simulink model "IEEE30_case"  (R2024b)
settings: Solver=FixedStepAuto  StartTime=0  StopTime=5  FixedStep=1e-7  RelTol=1e-3
values from neighbouring files (symbols this model uses):
  GFL_DFIG_7_C_bus = 0.08    [IEEE30_case_parameters.m]
  GFL_DFIG_7_D_mutual = 2.500000e+3    (= 2500)    [IEEE30_case_parameters.m]
  GFL_DFIG_7_f0 = 60    [IEEE30_case_parameters.m]
  GFL_DFIG_7_gPLLi = 3200    [IEEE30_case_parameters.m]
  GFL_DFIG_7_gPLLp = 650    [IEEE30_case_parameters.m]
  GFL_DFIG_7_H_WT = 0.4    [IEEE30_case_parameters.m]
  GFL_DFIG_7_Hg = 0.8    [IEEE30_case_parameters.m]
  GFL_DFIG_7_Igq_ref = 0    [IEEE30_case_parameters.m]
  GFL_DFIG_7_Ird_ref = 704.45696    [IEEE30_case_parameters.m]
  GFL_DFIG_7_KI_V = -300000    [IEEE30_case_parameters.m]
  GFL_DFIG_7_KP_V = -1000    [IEEE30_case_parameters.m]
  GFL_DFIG_7_Ksh = 1.254300e+4    (= 12543)    [IEEE30_case_parameters.m]
  GFL_DFIG_7_Lg = 0.000483    [IEEE30_case_parameters.m]
  GFL_DFIG_7_Lm_pu = 4    [IEEE30_case_parameters.m]
  GFL_DFIG_7_N = 100    [IEEE30_case_parameters.m]
  GFL_DFIG_7_p = 2    [IEEE30_case_parameters.m]
  GFL_DFIG_7_Pitch = 0    [IEEE30_case_parameters.m]
  GFL_DFIG_7_R = 44    [IEEE30_case_parameters.m]
  GFL_DFIG_7_Rg = 2.000000e-5    (= 2e-05)    [IEEE30_case_parameters.m]
  GFL_DFIG_7_rho = 1.225    [IEEE30_case_parameters.m]
  GFL_DFIG_7_rPLLi = 4500    [IEEE30_case_parameters.m]
  GFL_DFIG_7_rPLLp = 620    [IEEE30_case_parameters.m]
  GFL_DFIG_7_Rs_pu = 0.011    [IEEE30_case_parameters.m]
  GFL_DFIG_7_Sbase = 2.000000e+6    (= 2000000)    [IEEE30_case_parameters.m]
  GFL_DFIG_7_ugq_ref = 0    [IEEE30_case_parameters.m]
  GFL_DFIG_7_usd_ref = 0    [IEEE30_case_parameters.m]
  GFL_DFIG_7_Vbase = 690    [IEEE30_case_parameters.m]
  GFL_DFIG_7_Vdc_ref = 1200    [IEEE30_case_parameters.m]
  GFL_DFIG_7_wind = 12    [IEEE30_case_parameters.m]
  GFL_DFIG_7_wm_ref = 518.184209    [IEEE30_case_parameters.m]
  SG_D_13_D = 0.01056    [IEEE30_case_parameters.m]
  SG_D_13_EnableSaturation = 0    [IEEE30_case_parameters.m]
  SG_D_13_f0 = 60    [IEEE30_case_parameters.m]
  SG_D_13_H = 7.5    [IEEE30_case_parameters.m]
  SG_D_13_K_A = 20    [IEEE30_case_parameters.m]
  SG_D_13_K_E = 1.000000e+1    (= 10)    [IEEE30_case_parameters.m]
  SG_D_13_K_F = 2.363    [IEEE30_case_parameters.m]
  SG_D_13_K_s = 0.5    [IEEE30_case_parameters.m]
  SG_D_13_R_a = 0.001088    [IEEE30_case_parameters.m]
  SG_D_13_S_A = 1    [IEEE30_case_parameters.m]
  SG_D_13_S_B = 0.103    [IEEE30_case_parameters.m]
  SG_D_13_S_N = 10.659857    [IEEE30_case_parameters.m]
  SG_D_13_SpeedPara = 200    [IEEE30_case_parameters.m]
  SG_D_13_T_0 = 0.370163    [IEEE30_case_parameters.m]
  SG_D_13_T_1 = 0.3    [IEEE30_case_parameters.m]
  SG_D_13_T_2 = 0.05    [IEEE30_case_parameters.m]
  SG_D_13_T_3 = 0.02    [IEEE30_case_parameters.m]
  SG_D_13_T_4 = 0.005    [IEEE30_case_parameters.m]
  SG_D_13_T_A = 0.02    [IEEE30_case_parameters.m]
  SG_D_13_T_dd = 8.000000e+0    (= 8)    [IEEE30_case_parameters.m]
  SG_D_13_T_ddd = 0.04    [IEEE30_case_parameters.m]
  SG_D_13_T_E = 0.314    [IEEE30_case_parameters.m]
  SG_D_13_T_F = 0.35    [IEEE30_case_parameters.m]
  SG_D_13_T_qd = 0.8    [IEEE30_case_parameters.m]
  SG_D_13_T_qdd = 0.02    [IEEE30_case_parameters.m]
  SG_D_13_T_speed = 0.1    [IEEE30_case_parameters.m]
  SG_D_13_T_w = 0.5    [IEEE30_case_parameters.m]
  SG_D_13_V_ref = 1.696619    [IEEE30_case_parameters.m]
  SG_D_13_w_ref = 376.991118    [IEEE30_case_parameters.m]
  SG_D_13_x_d = 1.9    [IEEE30_case_parameters.m]
  SG_D_13_x_dd = 0.302    [IEEE30_case_parameters.m]
  SG_D_13_x_ddd = 0.204    [IEEE30_case_parameters.m]
  SG_D_13_x_l = 0.05    [IEEE30_case_parameters.m]
  SG_D_13_x_q = 1.3    [IEEE30_case_parameters.m]
  SG_D_13_x_qd = 0.5    [IEEE30_case_parameters.m]
  SG_D_13_x_qdd = 0.3    [IEEE30_case_parameters.m]
  SG_D_1_D = 0.01056    [IEEE30_case_parameters.m]
  SG_D_1_EnableSaturation = 0    [IEEE30_case_parameters.m]
  SG_D_1_f0 = 60    [IEEE30_case_parameters.m]
  SG_D_1_H = 7.5    [IEEE30_case_parameters.m]
  SG_D_1_K_A = 20    [IEEE30_case_parameters.m]
  SG_D_1_K_E = 1.000000e+1    (= 10)    [IEEE30_case_parameters.m]
  SG_D_1_K_F = 2.363    [IEEE30_case_parameters.m]
  SG_D_1_K_s = 0.5    [IEEE30_case_parameters.m]
  SG_D_1_R_a = 0.001088    [IEEE30_case_parameters.m]
  SG_D_1_S_A = 1    [IEEE30_case_parameters.m]
  SG_D_1_S_B = 0.103    [IEEE30_case_parameters.m]
  SG_D_1_S_N = 10.659857    [IEEE30_case_parameters.m]
  SG_D_1_SpeedPara = 200    [IEEE30_case_parameters.m]
  SG_D_1_T_0 = 0.259812    [IEEE30_case_parameters.m]
  SG_D_1_T_1 = 0.3    [IEEE30_case_parameters.m]
  SG_D_1_T_2 = 0.05    [IEEE30_case_parameters.m]
  SG_D_1_T_3 = 0.02    [IEEE30_case_parameters.m]
  SG_D_1_T_4 = 0.005    [IEEE30_case_parameters.m]
  SG_D_1_T_A = 0.02    [IEEE30_case_parameters.m]
  SG_D_1_T_dd = 8.000000e+0    (= 8)    [IEEE30_case_parameters.m]
  SG_D_1_T_ddd = 0.04    [IEEE30_case_parameters.m]
  SG_D_1_T_E = 0.314    [IEEE30_case_parameters.m]
  SG_D_1_T_F = 0.35    [IEEE30_case_parameters.m]
  SG_D_1_T_qd = 0.8    [IEEE30_case_parameters.m]
  SG_D_1_T_qdd = 0.02    [IEEE30_case_parameters.m]
  SG_D_1_T_speed = 0.1    [IEEE30_case_parameters.m]
  SG_D_1_T_w = 0.5    [IEEE30_case_parameters.m]
  SG_D_1_V_ref = 1.544107    [IEEE30_case_parameters.m]
  SG_D_1_w_ref = 376.991118    [IEEE30_case_parameters.m]
  SG_D_1_x_d = 1.9    [IEEE30_case_parameters.m]
  SG_D_1_x_dd = 0.302    [IEEE30_case_parameters.m]
  SG_D_1_x_ddd = 0.204    [IEEE30_case_parameters.m]
  SG_D_1_x_l = 0.05    [IEEE30_case_parameters.m]
  SG_D_1_x_q = 1.3    [IEEE30_case_parameters.m]
  SG_D_1_x_qd = 0.5    [IEEE30_case_parameters.m]
  SG_D_1_x_qdd = 0.3    [IEEE30_case_parameters.m]
  SG_D_22_D = 0.01056    [IEEE30_case_parameters.m]
  SG_D_22_EnableSaturation = 0    [IEEE30_case_parameters.m]
  SG_D_22_f0 = 60    [IEEE30_case_parameters.m]
  SG_D_22_H = 7.5    [IEEE30_case_parameters.m]
  SG_D_22_K_A = 20    [IEEE30_case_parameters.m]
  SG_D_22_K_E = 1.000000e+1    (= 10)    [IEEE30_case_parameters.m]
  SG_D_22_K_F = 2.363    [IEEE30_case_parameters.m]
  SG_D_22_K_s = 0.5    [IEEE30_case_parameters.m]
  SG_D_22_R_a = 0.001088    [IEEE30_case_parameters.m]
  SG_D_22_S_A = 1    [IEEE30_case_parameters.m]
  SG_D_22_S_B = 0.103    [IEEE30_case_parameters.m]
  SG_D_22_S_N = 10.659857    [IEEE30_case_parameters.m]
  SG_D_22_SpeedPara = 200    [IEEE30_case_parameters.m]
  SG_D_22_T_0 = 0.216121    [IEEE30_case_parameters.m]
  SG_D_22_T_1 = 0.3    [IEEE30_case_parameters.m]
  SG_D_22_T_2 = 0.05    [IEEE30_case_parameters.m]
  SG_D_22_T_3 = 0.02    [IEEE30_case_parameters.m]
  SG_D_22_T_4 = 0.005    [IEEE30_case_parameters.m]
  ... (+126 more)
(part 5 of 27)

== system IEEE30_case/AC_1/d_id_line_12_15_block ==
  note: d_id_line_12_15 in IEEE30_case
      | $376.991118430775\,\mathrm{iq}_{\mathrm{line},12,15}-202.995217616571\,\mathrm{id}_{\mathrm{line},12,15}+2899.93168023673\,\mathrm{vd}_{\mathrm{bus},12}-2899.93168023673\,\mathrm{vd}_{\mathrm{bus},15}$
      | Automatically generated on 2025-11-01 18:41:36 .
  State_id_line_12_15_19cb2 : Inport
  State_iq_line_12_15_08071 : Inport  Port=2
  State_vd_bus_12_a4ba8 : Inport  Port=3
  State_vd_bus_15_2851a : Inport  Port=4
  Add_1c604 : Sum
  Add_88b54 : Sum
  Constant_-202.995217616571_6ff68 : Constant  Value=-202.995217616571
  Constant_2899.93168023673_4202a : Constant  Value=2899.93168023673
  Constant_2899.93168023673_fe615 : Constant  Value=2899.93168023673
  Constant_376.991118430775_4d075 : Constant  Value=376.991118430775
  Product_04dd2 : Product
  Product_066f0 : Product
  Product_6a2b6 : Product
  Product_79b71 : Product
  Subtract_280ce : Sum  Inputs=+-
  Blockout_d_id_line_12_15_9a1c2 : Outport
  wires:
  State_id_line_12_15_19cb2/1 -> Product_04dd2/2
  Constant_-202.995217616571_6ff68/1 -> Product_04dd2/1
  Constant_376.991118430775_4d075/1 -> Product_79b71/1
  Product_6a2b6/1 -> Add_1c604/2
  Constant_2899.93168023673_fe615/1 -> Product_6a2b6/1
  State_iq_line_12_15_08071/1 -> Product_79b71/2
  Product_79b71/1 -> Add_88b54/2
  Product_04dd2/1 -> Add_88b54/1
  State_vd_bus_12_a4ba8/1 -> Product_6a2b6/2
  Add_88b54/1 -> Add_1c604/1
  Product_066f0/1 -> Subtract_280ce/2
  Constant_2899.93168023673_4202a/1 -> Product_066f0/1
  State_vd_bus_15_2851a/1 -> Product_066f0/2
  Add_1c604/1 -> Subtract_280ce/1
  Subtract_280ce/1 -> Blockout_d_id_line_12_15_9a1c2/1

== system IEEE30_case/AC_1/d_id_line_12_16_block ==
  note: d_id_line_12_16 in IEEE30_case
      | $376.991118430775\,\mathrm{iq}_{\mathrm{line},12,16}-169.646003293849\,\mathrm{id}_{\mathrm{line},12,16}+1884.95559215388\,\mathrm{vd}_{\mathrm{bus},12}-1884.95559215388\,\mathrm{vd}_{\mathrm{bus},16}$
      | Automatically generated on 2025-11-01 18:41:38 .
  State_id_line_12_16_8024a : Inport
  State_iq_line_12_16_288fb : Inport  Port=2
  State_vd_bus_12_31adb : Inport  Port=3
  State_vd_bus_16_dfe3f : Inport  Port=4
  Add_7fa9a : Sum
  Add_82f4b : Sum
  Constant_-169.646003293849_e986b : Constant  Value=-169.646003293849
  Constant_1884.95559215388_c1875 : Constant  Value=1884.95559215388
  Constant_1884.95559215388_da5ce : Constant  Value=1884.95559215388
  Constant_376.991118430775_e57b6 : Constant  Value=376.991118430775
  Product_08c30 : Product
  Product_0c215 : Product
  Product_538c2 : Product
  Product_ba034 : Product
  Subtract_28196 : Sum  Inputs=+-
  Blockout_d_id_line_12_16_004d6 : Outport
  wires:
  Constant_-169.646003293849_e986b/1 -> Product_08c30/1
  Constant_376.991118430775_e57b6/1 -> Product_538c2/1
  Product_538c2/1 -> Add_82f4b/2
  State_id_line_12_16_8024a/1 -> Product_08c30/2
  State_iq_line_12_16_288fb/1 -> Product_538c2/2
  Product_08c30/1 -> Add_82f4b/1
  Constant_1884.95559215388_c1875/1 -> Product_ba034/1
  State_vd_bus_12_31adb/1 -> Product_ba034/2
  Add_82f4b/1 -> Add_7fa9a/1
  Product_ba034/1 -> Add_7fa9a/2
  Product_0c215/1 -> Subtract_28196/2
  Constant_1884.95559215388_da5ce/1 -> Product_0c215/1
  State_vd_bus_16_dfe3f/1 -> Product_0c215/2
  Add_7fa9a/1 -> Subtract_28196/1
  Subtract_28196/1 -> Blockout_d_id_line_12_16_004d6/1

== system IEEE30_case/AC_1/d_id_line_14_15_block ==
  note: d_id_line_14_15 in IEEE30_case
      | $376.991118430775\,\mathrm{iq}_{\mathrm{line},14,15}-414.690230273853\,\mathrm{id}_{\mathrm{line},14,15}+1884.95559215388\,\mathrm{vd}_{\mathrm{bus},14}-1884.95559215388\,\mathrm{vd}_{\mathrm{bus},15}$
      | Automatically generated on 2025-11-01 18:41:40 .
  State_id_line_14_15_28cb1 : Inport
  State_iq_line_14_15_9579a : Inport  Port=2
  State_vd_bus_14_5ffe4 : Inport  Port=3
  State_vd_bus_15_c6d58 : Inport  Port=4
  Add_03647 : Sum
  Add_442a9 : Sum
  Constant_-414.690230273853_aa946 : Constant  Value=-414.690230273853
  Constant_1884.95559215388_3e1ac : Constant  Value=1884.95559215388
  Constant_1884.95559215388_7cbb8 : Constant  Value=1884.95559215388
  Constant_376.991118430775_5b540 : Constant  Value=376.991118430775
  Product_16522 : Product
  Product_81fd4 : Product
  Product_9c15a : Product
  Product_c85a0 : Product
  Subtract_fac3d : Sum  Inputs=+-
  Blockout_d_id_line_14_15_f4e19 : Outport
  wires:
  Product_c85a0/1 -> Add_03647/1
  Constant_-414.690230273853_aa946/1 -> Product_c85a0/1
  State_id_line_14_15_28cb1/1 -> Product_c85a0/2
  Constant_376.991118430775_5b540/1 -> Product_16522/1
  Product_16522/1 -> Add_03647/2
  State_iq_line_14_15_9579a/1 -> Product_16522/2
  Product_9c15a/1 -> Add_442a9/2
  Constant_1884.95559215388_3e1ac/1 -> Product_9c15a/1
  State_vd_bus_14_5ffe4/1 -> Product_9c15a/2
  Add_03647/1 -> Add_442a9/1
  Product_81fd4/1 -> Subtract_fac3d/2
  Constant_1884.95559215388_7cbb8/1 -> Product_81fd4/1
  State_vd_bus_15_c6d58/1 -> Product_81fd4/2
  Add_442a9/1 -> Subtract_fac3d/1
  Subtract_fac3d/1 -> Blockout_d_id_line_14_15_f4e19/1

== system IEEE30_case/AC_1/d_id_line_15_18_block ==
  note: d_id_line_15_18 in IEEE30_case
      | $376.991118430775\,\mathrm{iq}_{\mathrm{line},15,18}-188.495559215388\,\mathrm{id}_{\mathrm{line},15,18}+1713.59599286716\,\mathrm{vd}_{\mathrm{bus},15}-1713.59599286716\,\mathrm{vd}_{\mathrm{bus},18}$
      | Automatically generated on 2025-11-01 18:41:45 .
  State_id_line_15_18_9ff35 : Inport
  State_iq_line_15_18_872e9 : Inport  Port=2
  State_vd_bus_15_67b4c : Inport  Port=3
  State_vd_bus_18_e7afb : Inport  Port=4
  Add_4abb7 : Sum
  Add_ea80a : Sum
  Constant_-188.495559215388_eae43 : Constant  Value=-188.495559215388
  Constant_1713.59599286716_37fdf : Constant  Value=1713.59599286716
  Constant_1713.59599286716_e4c6f : Constant  Value=1713.59599286716
  Constant_376.991118430775_f78d8 : Constant  Value=376.991118430775
  Product_a3e74 : Product
  Product_c991e : Product
  Product_e914a : Product
  Product_ea7c3 : Product
  Subtract_e5fa3 : Sum  Inputs=+-
  Blockout_d_id_line_15_18_32fdd : Outport
  wires:
  Constant_-188.495559215388_eae43/1 -> Product_ea7c3/1
  Constant_376.991118430775_f78d8/1 -> Product_a3e74/1
  State_id_line_15_18_9ff35/1 -> Product_ea7c3/2
  Product_a3e74/1 -> Add_ea80a/2
  State_iq_line_15_18_872e9/1 -> Product_a3e74/2
  Product_ea7c3/1 -> Add_ea80a/1
  State_vd_bus_15_67b4c/1 -> Product_c991e/2
  Product_c991e/1 -> Add_4abb7/2
  Constant_1713.59599286716_e4c6f/1 -> Product_c991e/1
  Add_ea80a/1 -> Add_4abb7/1
  Product_e914a/1 -> Subtract_e5fa3/2
  Constant_1713.59599286716_37fdf/1 -> Product_e914a/1
  State_vd_bus_18_e7afb/1 -> Product_e914a/2
  Add_4abb7/1 -> Subtract_e5fa3/1
  Subtract_e5fa3/1 -> Blockout_d_id_line_15_18_32fdd/1

== system IEEE30_case/AC_1/d_id_line_15_23_block ==
  note: d_id_line_15_23 in IEEE30_case
      | $376.991118430775\,\mathrm{iq}_{\mathrm{line},15,23}-188.495559215388\,\mathrm{id}_{\mathrm{line},15,23}+1884.95559215388\,\mathrm{vd}_{\mathrm{bus},15}-1884.95559215388\,\mathrm{vd}_{\mathrm{bus},23}$
      | Automatically generated on 2025-11-01 18:42:03 .
  State_id_line_15_23_5b9f7 : Inport
  State_iq_line_15_23_b33ff : Inport  Port=2
  State_vd_bus_15_742a0 : Inport  Port=3
  State_vd_bus_23_ce9b8 : Inport  Port=4
  Add_304c8 : Sum
  Add_d6195 : Sum
  Constant_-188.495559215388_5b43b : Constant  Value=-188.495559215388
  Constant_1884.95559215388_346b1 : Constant  Value=1884.95559215388
  Constant_1884.95559215388_64cf3 : Constant  Value=1884.95559215388
  Constant_376.991118430775_82cf8 : Constant  Value=376.991118430775
  Product_18461 : Product
  Product_35b29 : Product
  Product_4bfc7 : Product
  Product_954db : Product
  Subtract_3f90f : Sum  Inputs=+-
  Blockout_d_id_line_15_23_c2a70 : Outport
  wires:
  Constant_-188.495559215388_5b43b/1 -> Product_35b29/1
  State_id_line_15_23_5b9f7/1 -> Product_35b29/2
  Constant_376.991118430775_82cf8/1 -> Product_4bfc7/1
  State_iq_line_15_23_b33ff/1 -> Product_4bfc7/2
  Product_4bfc7/1 -> Add_304c8/2
  Product_35b29/1 -> Add_304c8/1
  Product_18461/1 -> Add_d6195/2
  Constant_1884.95559215388_64cf3/1 -> Product_18461/1
  State_vd_bus_15_742a0/1 -> Product_18461/2
  Add_304c8/1 -> Add_d6195/1
  Product_954db/1 -> Subtract_3f90f/2
  Constant_1884.95559215388_346b1/1 -> Product_954db/1
  State_vd_bus_23_ce9b8/1 -> Product_954db/2
  Add_d6195/1 -> Subtract_3f90f/1
  Subtract_3f90f/1 -> Blockout_d_id_line_15_23_c2a70/1

== system IEEE30_case/AC_1/d_id_line_16_17_block ==
  note: d_id_line_16_17 in IEEE30_case
      | $376.991118430775\,\mathrm{iq}_{\mathrm{line},16,17}-158.733102497168\,\mathrm{id}_{\mathrm{line},16,17}+1984.16378121461\,\mathrm{vd}_{\mathrm{bus},16}-1984.16378121461\,\mathrm{vd}_{\mathrm{bus},17}$
      | Automatically generated on 2025-11-01 18:41:43 .
  State_id_line_16_17_5c8bf : Inport
  State_iq_line_16_17_49d5c : Inport  Port=2
  State_vd_bus_16_c102f : Inport  Port=3
  State_vd_bus_17_81d16 : Inport  Port=4
  Add_48fb3 : Sum
  Add_527f8 : Sum
  Constant_-158.733102497168_b2c29 : Constant  Value=-158.733102497168
  Constant_1984.16378121461_03e4f : Constant  Value=1984.16378121461
  Constant_1984.16378121461_7c6ef : Constant  Value=1984.16378121461
  Constant_376.991118430775_1e0c9 : Constant  Value=376.991118430775
  Product_01cb9 : Product
  Product_0d51e : Product
  Product_5ed86 : Product
  Product_f72dc : Product
  Subtract_cb5b6 : Sum  Inputs=+-
  Blockout_d_id_line_16_17_1cf66 : Outport
  wires:
  Constant_-158.733102497168_b2c29/1 -> Product_f72dc/1
  Constant_376.991118430775_1e0c9/1 -> Product_01cb9/1
  Product_01cb9/1 -> Add_48fb3/2
  Product_f72dc/1 -> Add_48fb3/1
  State_id_line_16_17_5c8bf/1 -> Product_f72dc/2
  Product_0d51e/1 -> Add_527f8/2
  Constant_1984.16378121461_03e4f/1 -> Product_0d51e/1
  State_iq_line_16_17_49d5c/1 -> Product_01cb9/2
  State_vd_bus_16_c102f/1 -> Product_0d51e/2
  Add_48fb3/1 -> Add_527f8/1
  Constant_1984.16378121461_7c6ef/1 -> Product_5ed86/1
  Add_527f8/1 -> Subtract_cb5b6/1
  State_vd_bus_17_81d16/1 -> Product_5ed86/2
  Product_5ed86/1 -> Subtract_cb5b6/2
  Subtract_cb5b6/1 -> Blockout_d_id_line_16_17_1cf66/1

== system IEEE30_case/AC_1/d_id_line_18_19_block ==
  note: d_id_line_18_19 in IEEE30_case
      | $376.991118430775\,\mathrm{iq}_{\mathrm{line},18,19}-173.995900814204\,\mathrm{id}_{\mathrm{line},18,19}+2899.93168023673\,\mathrm{vd}_{\mathrm{bus},18}-2899.93168023673\,\mathrm{vd}_{\mathrm{bus},19}$
      | Automatically generated on 2025-11-01 18:41:47 .
  State_id_line_18_19_ee31e : Inport
  State_iq_line_18_19_bad0a : Inport  Port=2
  State_vd_bus_18_26e57 : Inport  Port=3
  State_vd_bus_19_37873 : Inport  Port=4
  Add_0bb69 : Sum
  Add_79b81 : Sum
  Constant_-173.995900814204_e40f3 : Constant  Value=-173.995900814204
  Constant_2899.93168023673_2d509 : Constant  Value=2899.93168023673
  Constant_2899.93168023673_80d84 : Constant  Value=2899.93168023673
  Constant_376.991118430775_81f31 : Constant  Value=376.991118430775
  Product_a93df : Product
  Product_b05af : Product
  Product_ca76e : Product
  Product_e4da4 : Product
  Subtract_630ad : Sum  Inputs=+-
  Blockout_d_id_line_18_19_39807 : Outport
  wires:
  State_id_line_18_19_ee31e/1 -> Product_a93df/2
  Constant_-173.995900814204_e40f3/1 -> Product_a93df/1
  Constant_376.991118430775_81f31/1 -> Product_ca76e/1
  Product_ca76e/1 -> Add_0bb69/2
  State_iq_line_18_19_bad0a/1 -> Product_ca76e/2
  Product_a93df/1 -> Add_0bb69/1
  Add_0bb69/1 -> Add_79b81/1
  Constant_2899.93168023673_80d84/1 -> Product_b05af/1
  State_vd_bus_18_26e57/1 -> Product_b05af/2
  Product_b05af/1 -> Add_79b81/2
  Product_e4da4/1 -> Subtract_630ad/2
  Constant_2899.93168023673_2d509/1 -> Product_e4da4/1
  State_vd_bus_19_37873/1 -> Product_e4da4/2
  Add_79b81/1 -> Subtract_630ad/1
  Subtract_630ad/1 -> Blockout_d_id_line_18_19_39807/1

== system IEEE30_case/AC_1/d_id_line_19_20_block ==
  note: d_id_line_19_20 in IEEE30_case
      | $376.991118430775\,\mathrm{iq}_{\mathrm{line},19,20}-161.567622184618\,\mathrm{id}_{\mathrm{line},19,20}+5385.58740615393\,\mathrm{vd}_{\mathrm{bus},19}-5385.58740615393\,\mathrm{vd}_{\mathrm{bus},20}$
      | Automatically generated on 2025-11-01 18:41:49 .
  State_id_line_19_20_52ad5 : Inport
  State_iq_line_19_20_aecba : Inport  Port=2
  State_vd_bus_19_720ac : Inport  Port=3
  State_vd_bus_20_fc360 : Inport  Port=4
  Add_85617 : Sum
  Add_b55b6 : Sum
  Constant_-161.567622184618_669a2 : Constant  Value=-161.567622184618
  Constant_376.991118430775_79d8f : Constant  Value=376.991118430775
  Constant_5385.58740615393_4a1b5 : Constant  Value=5385.58740615393
  Constant_5385.58740615393_9f343 : Constant  Value=5385.58740615393
  Product_21136 : Product
  Product_39dca : Product
  Product_62d92 : Product
  Product_79959 : Product
  Subtract_e7c18 : Sum  Inputs=+-
  Blockout_d_id_line_19_20_50907 : Outport
  wires:
  State_vd_bus_19_720ac/1 -> Product_79959/2
  Constant_-161.567622184618_669a2/1 -> Product_21136/1
  Product_79959/1 -> Add_85617/2
  Constant_5385.58740615393_9f343/1 -> Product_79959/1
  Subtract_e7c18/1 -> Blockout_d_id_line_19_20_50907/1
  State_id_line_19_20_52ad5/1 -> Product_21136/2
  Constant_376.991118430775_79d8f/1 -> Product_39dca/1
  Product_39dca/1 -> Add_b55b6/2
  State_iq_line_19_20_aecba/1 -> Product_39dca/2
  Product_21136/1 -> Add_b55b6/1
  Add_b55b6/1 -> Add_85617/1
  Product_62d92/1 -> Subtract_e7c18/2
  Constant_5385.58740615393_4a1b5/1 -> Product_62d92/1
  State_vd_bus_20_fc360/1 -> Product_62d92/2
  Add_85617/1 -> Subtract_e7c18/1

== system IEEE30_case/AC_1/d_id_line_1_2_block ==
  note: d_id_line_1_2 in IEEE30_case
      | $376.991118430775\,\mathrm{iq}_{\mathrm{line},1,2}-125.663706143592\,\mathrm{id}_{\mathrm{line},1,2}+6283.18530717959\,\mathrm{vd}_{\mathrm{bus},1}-6283.18530717959\,\mathrm{vd}_{\mathrm{bus},2}$
      | Automatically generated on 2025-11-01 18:40:56 .
  State_id_line_1_2_ffdd4 : Inport
  State_iq_line_1_2_034b5 : Inport  Port=2
  State_vd_bus_1_c4c37 : Inport  Port=3
  State_vd_bus_2_3fb4b : Inport  Port=4
  Add_2f17b : Sum
  Add_58b2b : Sum
  Constant_-125.663706143592_1505d : Constant  Value=-125.663706143592
  Constant_376.991118430775_520bb : Constant  Value=376.991118430775
  Constant_6283.18530717959_4c671 : Constant  Value=6283.18530717959
  Constant_6283.18530717959_8a0e7 : Constant  Value=6283.18530717959
  Product_36a67 : Product
  Product_59a0b : Product
  Product_b8331 : Product
  Product_bf9d6 : Product
  Subtract_e7e69 : Sum  Inputs=+-
  Blockout_d_id_line_1_2_c33ff : Outport
  wires:
  Constant_-125.663706143592_1505d/1 -> Product_59a0b/1
  Product_59a0b/1 -> Add_58b2b/1
  State_id_line_1_2_ffdd4/1 -> Product_59a0b/2
  Constant_376.991118430775_520bb/1 -> Product_b8331/1
  Product_b8331/1 -> Add_58b2b/2
  State_iq_line_1_2_034b5/1 -> Product_b8331/2
  Constant_6283.18530717959_8a0e7/1 -> Product_bf9d6/1
  State_vd_bus_1_c4c37/1 -> Product_bf9d6/2
  Add_58b2b/1 -> Add_2f17b/1
  Product_bf9d6/1 -> Add_2f17b/2
  Product_36a67/1 -> Subtract_e7e69/2
  Constant_6283.18530717959_4c671/1 -> Product_36a67/1
  State_vd_bus_2_3fb4b/1 -> Product_36a67/2
  Add_2f17b/1 -> Subtract_e7e69/1
  Subtract_e7e69/1 -> Blockout_d_id_line_1_2_c33ff/1

== system IEEE30_case/AC_1/d_id_line_1_3_block ==
  note: d_id_line_1_3 in IEEE30_case
      | $376.991118430775\,\mathrm{iq}_{\mathrm{line},1,3}-99.2081890607303\,\mathrm{id}_{\mathrm{line},1,3}+1984.16378121461\,\mathrm{vd}_{\mathrm{bus},1}-1984.16378121461\,\mathrm{vd}_{\mathrm{bus},3}$
      | Automatically generated on 2025-11-01 18:40:59 .
  State_id_line_1_3_6eb6f : Inport
  State_iq_line_1_3_e0dcf : Inport  Port=2
  State_vd_bus_1_5ec44 : Inport  Port=3
  State_vd_bus_3_137a9 : Inport  Port=4
  Add_ca1fc : Sum
  Add_ef84b : Sum
  Constant_-99.2081890607303_6888c : Constant  Value=-99.2081890607303
  Constant_1984.16378121461_ea0d7 : Constant  Value=1984.16378121461
  Constant_1984.16378121461_ffcf3 : Constant  Value=1984.16378121461
  Constant_376.991118430775_83195 : Constant  Value=376.991118430775
  Product_145be : Product
  Product_4bd44 : Product
  Product_9bf79 : Product
  Product_e1655 : Product
  Subtract_92bee : Sum  Inputs=+-
  Blockout_d_id_line_1_3_0fd49 : Outport
  wires:
  State_vd_bus_1_5ec44/1 -> Product_4bd44/2
  Constant_-99.2081890607303_6888c/1 -> Product_9bf79/1
  Subtract_92bee/1 -> Blockout_d_id_line_1_3_0fd49/1
  Product_4bd44/1 -> Add_ca1fc/2
  Constant_1984.16378121461_ea0d7/1 -> Product_4bd44/1
  State_id_line_1_3_6eb6f/1 -> Product_9bf79/2
  Constant_376.991118430775_83195/1 -> Product_145be/1
  Product_145be/1 -> Add_ef84b/2
  State_iq_line_1_3_e0dcf/1 -> Product_145be/2
  Product_9bf79/1 -> Add_ef84b/1
  Add_ef84b/1 -> Add_ca1fc/1
  Product_e1655/1 -> Subtract_92bee/2
  Constant_1984.16378121461_ffcf3/1 -> Product_e1655/1
  State_vd_bus_3_137a9/1 -> Product_e1655/2
  Add_ca1fc/1 -> Subtract_92bee/1

== system IEEE30_case/AC_1/d_id_line_21_22_block ==
  note: d_id_line_21_22 in IEEE30_case
      | $376.991118430775\,\mathrm{iq}_{\mathrm{line},21,22}-188.495559215388\,\mathrm{id}_{\mathrm{line},21,22}+18849.5559215388\,\mathrm{vd}_{\mathrm{bus},21}-18849.5559215388\,\mathrm{vd}_{\mathrm{bus},22}$
      | Automatically generated on 2025-11-01 18:42:01 .
  State_id_line_21_22_e74c3 : Inport
  State_iq_line_21_22_c44a2 : Inport  Port=2
  State_vd_bus_21_3bbf1 : Inport  Port=3
  State_vd_bus_22_0f9f9 : Inport  Port=4
  Add_a94fd : Sum
  Add_d5fe7 : Sum
  Constant_-188.495559215388_66e3d : Constant  Value=-188.495559215388
  Constant_18849.5559215388_40e67 : Constant  Value=18849.5559215388
  Constant_18849.5559215388_ea422 : Constant  Value=18849.5559215388
  Constant_376.991118430775_2fe7b : Constant  Value=376.991118430775
  Product_43b02 : Product
  Product_6b97b : Product
  Product_9d2a6 : Product
  Product_a7a63 : Product
  Subtract_3876f : Sum  Inputs=+-
  Blockout_d_id_line_21_22_f50b1 : Outport
  wires:
  Constant_-188.495559215388_66e3d/1 -> Product_9d2a6/1
  State_vd_bus_21_3bbf1/1 -> Product_a7a63/2
  Subtract_3876f/1 -> Blockout_d_id_line_21_22_f50b1/1
  Product_a7a63/1 -> Add_d5fe7/2
  State_id_line_21_22_e74c3/1 -> Product_9d2a6/2
  Constant_18849.5559215388_40e67/1 -> Product_a7a63/1
  Product_9d2a6/1 -> Add_a94fd/1
  Constant_376.991118430775_2fe7b/1 -> Product_6b97b/1
  Product_6b97b/1 -> Add_a94fd/2
  State_iq_line_21_22_c44a2/1 -> Product_6b97b/2
  Add_a94fd/1 -> Add_d5fe7/1
  Constant_18849.5559215388_ea422/1 -> Product_43b02/1
  State_vd_bus_22_0f9f9/1 -> Product_43b02/2
  Add_d5fe7/1 -> Subtract_3876f/1
  Product_43b02/1 -> Subtract_3876f/2

== system IEEE30_case/AC_1/d_id_line_22_24_block ==
  note: d_id_line_22_24 in IEEE30_case
      | $376.991118430775\,\mathrm{iq}_{\mathrm{line},22,24}-251.327412287183\,\mathrm{id}_{\mathrm{line},22,24}+2094.39510239319\,\mathrm{vd}_{\mathrm{bus},22}-2094.39510239319\,\mathrm{vd}_{\mathrm{bus},24}$
      | Automatically generated on 2025-11-01 18:42:06 .
  State_id_line_22_24_bf52a : Inport
  State_iq_line_22_24_ef354 : Inport  Port=2
  State_vd_bus_22_6ca17 : Inport  Port=3
  State_vd_bus_24_440b0 : Inport  Port=4
  Add_a8bef : Sum
  Add_a9ee4 : Sum
  Constant_-251.327412287183_ec60e : Constant  Value=-251.327412287183
  Constant_2094.39510239319_47fe7 : Constant  Value=2094.39510239319
  Constant_2094.39510239319_cffec : Constant  Value=2094.39510239319
  Constant_376.991118430775_92cc2 : Constant  Value=376.991118430775
  Product_1b5e0 : Product
  Product_bae76 : Product
  Product_d00f9 : Product
  Product_d2185 : Product
  Subtract_2874d : Sum  Inputs=+-
  Blockout_d_id_line_22_24_ad4cf : Outport
  wires:
  Constant_-251.327412287183_ec60e/1 -> Product_1b5e0/1
  State_id_line_22_24_bf52a/1 -> Product_1b5e0/2
  Add_a8bef/1 -> Add_a9ee4/1
  Constant_376.991118430775_92cc2/1 -> Product_bae76/1
  Product_bae76/1 -> Add_a8bef/2
  State_iq_line_22_24_ef354/1 -> Product_bae76/2
  Product_1b5e0/1 -> Add_a8bef/1
  Constant_2094.39510239319_cffec/1 -> Product_d2185/1
  State_vd_bus_22_6ca17/1 -> Product_d2185/2
  Product_d2185/1 -> Add_a9ee4/2
  Product_d00f9/1 -> Subtract_2874d/2
  Constant_2094.39510239319_47fe7/1 -> Product_d00f9/1
  State_vd_bus_24_440b0/1 -> Product_d00f9/2
  Add_a9ee4/1 -> Subtract_2874d/1
  Subtract_2874d/1 -> Blockout_d_id_line_22_24_ad4cf/1

== system IEEE30_case/AC_1/d_id_line_23_24_block ==
  note: d_id_line_23_24 in IEEE30_case
      | $376.991118430775\,\mathrm{iq}_{\mathrm{line},23,24}-181.51424220741\,\mathrm{id}_{\mathrm{line},23,24}+1396.26340159546\,\mathrm{vd}_{\mathrm{bus},23}-1396.26340159546\,\mathrm{vd}_{\mathrm{bus},24}$
      | Automatically generated on 2025-11-01 18:42:08 .
  State_id_line_23_24_64227 : Inport
  State_iq_line_23_24_865cb : Inport  Port=2
  State_vd_bus_23_dd709 : Inport  Port=3
  State_vd_bus_24_85dda : Inport  Port=4
  Add_23eca : Sum
  Add_fdfa4 : Sum
  Constant_-181.51424220741_90a38 : Constant  Value=-181.51424220741
  Constant_1396.26340159546_003fb : Constant  Value=1396.26340159546
  Constant_1396.26340159546_e0537 : Constant  Value=1396.26340159546
  Constant_376.991118430775_42dc1 : Constant  Value=376.991118430775
  Product_18a24 : Product
  Product_23684 : Product
  Product_24cc1 : Product
  Product_434d9 : Product
  Subtract_28be3 : Sum  Inputs=+-
  Blockout_d_id_line_23_24_092ff : Outport
  wires:
  State_vd_bus_23_dd709/1 -> Product_434d9/2
  Constant_-181.51424220741_90a38/1 -> Product_23684/1
  Product_434d9/1 -> Add_23eca/2
  Constant_1396.26340159546_e0537/1 -> Product_434d9/1
  State_id_line_23_24_64227/1 -> Product_23684/2
  Constant_376.991118430775_42dc1/1 -> Product_24cc1/1
  Product_24cc1/1 -> Add_fdfa4/2
  State_iq_line_23_24_865cb/1 -> Product_24cc1/2
  Product_23684/1 -> Add_fdfa4/1
  Add_fdfa4/1 -> Add_23eca/1
  Product_18a24/1 -> Subtract_28be3/2
  Constant_1396.26340159546_003fb/1 -> Product_18a24/1
  State_vd_bus_24_85dda/1 -> Product_18a24/2
  Add_23eca/1 -> Subtract_28be3/1
  Subtract_28be3/1 -> Blockout_d_id_line_23_24_092ff/1

== system IEEE30_case/AC_1/d_id_line_24_25_block ==
  note: d_id_line_24_25 in IEEE30_case
      | $376.991118430775\,\mathrm{iq}_{\mathrm{line},24,25}-217.05549242984\,\mathrm{id}_{\mathrm{line},24,25}+1142.39732857811\,\mathrm{vd}_{\mathrm{bus},24}-1142.39732857811\,\mathrm{vd}_{\mathrm{bus},25}$
      | Automatically generated on 2025-11-01 18:42:11 .
  State_id_line_24_25_f5b6e : Inport
  State_iq_line_24_25_5d4c8 : Inport  Port=2
  State_vd_bus_24_6e200 : Inport  Port=3
  State_vd_bus_25_6942f : Inport  Port=4
  Add_1fbfb : Sum
  Add_382b1 : Sum
  Constant_-217.05549242984_ac25d : Constant  Value=-217.05549242984
  Constant_1142.39732857811_1b4c6 : Constant  Value=1142.39732857811
  Constant_1142.39732857811_ca533 : Constant  Value=1142.39732857811
  Constant_376.991118430775_90553 : Constant  Value=376.991118430775
  Product_0c925 : Product
  Product_31d8e : Product
  Product_5608f : Product
  Product_b42c2 : Product
  Subtract_db9f9 : Sum  Inputs=+-
  Blockout_d_id_line_24_25_64f9d : Outport
  wires:
  Constant_-217.05549242984_ac25d/1 -> Product_5608f/1
  Constant_376.991118430775_90553/1 -> Product_0c925/1
  Product_0c925/1 -> Add_382b1/2
  Product_5608f/1 -> Add_382b1/1
  State_id_line_24_25_f5b6e/1 -> Product_5608f/2
  State_iq_line_24_25_5d4c8/1 -> Product_0c925/2
  Product_31d8e/1 -> Add_1fbfb/2
  Constant_1142.39732857811_1b4c6/1 -> Product_31d8e/1
  State_vd_bus_24_6e200/1 -> Product_31d8e/2
  Add_382b1/1 -> Add_1fbfb/1
  Constant_1142.39732857811_ca533/1 -> Product_b42c2/1
  State_vd_bus_25_6942f/1 -> Product_b42c2/2
  Add_1fbfb/1 -> Subtract_db9f9/1
  Product_b42c2/1 -> Subtract_db9f9/2
  Subtract_db9f9/1 -> Blockout_d_id_line_24_25_64f9d/1

== system IEEE30_case/AC_1/d_id_line_25_26_block ==
  note: d_id_line_25_26 in IEEE30_case
      | $376.991118430775\,\mathrm{iq}_{\mathrm{line},25,26}-248.020472651826\,\mathrm{id}_{\mathrm{line},25,26}+992.081890607303\,\mathrm{vd}_{\mathrm{bus},25}-992.081890607303\,\mathrm{vd}_{\mathrm{bus},26}$
      | Automatically generated on 2025-11-01 18:42:13 .
  State_id_line_25_26_99f78 : Inport
  State_iq_line_25_26_dac95 : Inport  Port=2
  State_vd_bus_25_d2af0 : Inport  Port=3
  State_vd_bus_26_fc271 : Inport  Port=4
  Add_4cd81 : Sum
  Add_97c72 : Sum
  Constant_-248.020472651826_9bf90 : Constant  Value=-248.020472651826
  Constant_376.991118430775_7dac7 : Constant  Value=376.991118430775
  Constant_992.081890607303_5a77a : Constant  Value=992.081890607303
  Constant_992.081890607303_db759 : Constant  Value=992.081890607303
  Product_58962 : Product
  Product_6b49c : Product
  Product_95729 : Product
  Product_c1dd1 : Product
  Subtract_1f94d : Sum  Inputs=+-
  Blockout_d_id_line_25_26_a039c : Outport
  wires:
  Constant_-248.020472651826_9bf90/1 -> Product_95729/1
  State_id_line_25_26_99f78/1 -> Product_95729/2
  Constant_376.991118430775_7dac7/1 -> Product_6b49c/1
  State_iq_line_25_26_dac95/1 -> Product_6b49c/2
  Product_95729/1 -> Add_97c72/1
  Product_6b49c/1 -> Add_97c72/2
  State_vd_bus_25_d2af0/1 -> Product_58962/2
  Product_58962/1 -> Add_4cd81/2
  Constant_992.081890607303_db759/1 -> Product_58962/1
  Add_97c72/1 -> Add_4cd81/1
  Product_c1dd1/1 -> Subtract_1f94d/2
  Constant_992.081890607303_5a77a/1 -> Product_c1dd1/1
  State_vd_bus_26_fc271/1 -> Product_c1dd1/2
  Add_4cd81/1 -> Subtract_1f94d/1
  Subtract_1f94d/1 -> Blockout_d_id_line_25_26_a039c/1

== system IEEE30_case/AC_1/d_id_line_25_27_block ==
  note: d_id_line_25_27 in IEEE30_case
      | $376.991118430775\,\mathrm{iq}_{\mathrm{line},25,27}-197.471538225644\,\mathrm{id}_{\mathrm{line},25,27}+1795.19580205131\,\mathrm{vd}_{\mathrm{bus},25}-1795.19580205131\,\mathrm{vd}_{\mathrm{bus},27}$
      | Automatically generated on 2025-11-01 18:42:16 .
  State_id_line_25_27_be6b9 : Inport
  State_iq_line_25_27_73a3b : Inport  Port=2
  State_vd_bus_25_03d67 : Inport  Port=3
  State_vd_bus_27_199bb : Inport  Port=4
  Add_7b76b : Sum
  Add_9d516 : Sum
  Constant_-197.471538225644_cb02e : Constant  Value=-197.471538225644
  Constant_1795.19580205131_62d20 : Constant  Value=1795.19580205131
  Constant_1795.19580205131_e4b78 : Constant  Value=1795.19580205131
  Constant_376.991118430775_f50ac : Constant  Value=376.991118430775
  Product_694c8 : Product
  Product_a3ebe : Product
  Product_f7b67 : Product
  Product_fa67b : Product
  Subtract_f2c85 : Sum  Inputs=+-
  Blockout_d_id_line_25_27_d028e : Outport
  wires:
  State_id_line_25_27_be6b9/1 -> Product_f7b67/2
  Constant_-197.471538225644_cb02e/1 -> Product_f7b67/1
  Constant_376.991118430775_f50ac/1 -> Product_fa67b/1
  Product_fa67b/1 -> Add_9d516/2
  State_iq_line_25_27_73a3b/1 -> Product_fa67b/2
  Product_f7b67/1 -> Add_9d516/1
  Constant_1795.19580205131_e4b78/1 -> Product_a3ebe/1
  State_vd_bus_25_03d67/1 -> Product_a3ebe/2
  Add_9d516/1 -> Add_7b76b/1
  Product_a3ebe/1 -> Add_7b76b/2
  Product_694c8/1 -> Subtract_f2c85/2
  Constant_1795.19580205131_62d20/1 -> Product_694c8/1
  State_vd_bus_27_199bb/1 -> Product_694c8/2
  Add_7b76b/1 -> Subtract_f2c85/1
  Subtract_f2c85/1 -> Blockout_d_id_line_25_27_d028e/1

== system IEEE30_case/AC_1/d_id_line_27_29_block ==
  note: d_id_line_27_29 in IEEE30_case
      | $376.991118430775\,\mathrm{iq}_{\mathrm{line},27,29}-197.471538225644\,\mathrm{id}_{\mathrm{line},27,29}+897.597901025655\,\mathrm{vd}_{\mathrm{bus},27}-897.597901025655\,\mathrm{vd}_{\mathrm{bus},29}$
      | Automatically generated on 2025-11-01 18:42:20 .
  State_id_line_27_29_5dcac : Inport
  State_iq_line_27_29_70df7 : Inport  Port=2
  State_vd_bus_27_91239 : Inport  Port=3
  State_vd_bus_29_a9de4 : Inport  Port=4
  Add_8ce4c : Sum
  Add_f6eea : Sum
  Constant_-197.471538225644_0eb6a : Constant  Value=-197.471538225644
  Constant_376.991118430775_9e213 : Constant  Value=376.991118430775
  Constant_897.597901025655_877d6 : Constant  Value=897.597901025655
  Constant_897.597901025655_fe40e : Constant  Value=897.597901025655
  Product_30f4b : Product
  Product_3ac2a : Product
  Product_aa3fd : Product
  Product_ed83f : Product
  Subtract_d9a38 : Sum  Inputs=+-
  Blockout_d_id_line_27_29_5ee71 : Outport
  wires:
  State_vd_bus_27_91239/1 -> Product_3ac2a/2
  Constant_-197.471538225644_0eb6a/1 -> Product_30f4b/1
  Product_3ac2a/1 -> Add_8ce4c/2
  Constant_897.597901025655_fe40e/1 -> Product_3ac2a/1
  State_id_line_27_29_5dcac/1 -> Product_30f4b/2
  Constant_376.991118430775_9e213/1 -> Product_ed83f/1
  Product_ed83f/1 -> Add_f6eea/2
  State_iq_line_27_29_70df7/1 -> Product_ed83f/2
  Product_30f4b/1 -> Add_f6eea/1
  Add_f6eea/1 -> Add_8ce4c/1
  Product_aa3fd/1 -> Subtract_d9a38/2
  Constant_897.597901025655_877d6/1 -> Product_aa3fd/1
  State_vd_bus_29_a9de4/1 -> Product_aa3fd/2
  Add_8ce4c/1 -> Subtract_d9a38/1
  Subtract_d9a38/1 -> Blockout_d_id_line_27_29_5ee71/1

== system IEEE30_case/AC_1/d_id_line_27_30_block ==
  note: d_id_line_27_30 in IEEE30_case
      | $376.991118430775\,\mathrm{iq}_{\mathrm{line},27,30}-201.061929829747\,\mathrm{id}_{\mathrm{line},27,30}+628.318530717959\,\mathrm{vd}_{\mathrm{bus},27}-628.318530717959\,\mathrm{vd}_{\mathrm{bus},30}$
      | Automatically generated on 2025-11-01 18:42:22 .
  State_id_line_27_30_d82b5 : Inport
  State_iq_line_27_30_37807 : Inport  Port=2
  State_vd_bus_27_614b7 : Inport  Port=3
  State_vd_bus_30_fc433 : Inport  Port=4
  Add_96799 : Sum
  Add_97ca2 : Sum
  Constant_-201.061929829747_e8334 : Constant  Value=-201.061929829747
  Constant_376.991118430775_f2cd8 : Constant  Value=376.991118430775
  Constant_628.318530717959_93a50 : Constant  Value=628.318530717959
  Constant_628.318530717959_fb4b7 : Constant  Value=628.318530717959
  Product_1a1ae : Product
  Product_1c8cb : Product
  Product_7e1c1 : Product
  Product_cd5ec : Product
  Subtract_78c91 : Sum  Inputs=+-
  Blockout_d_id_line_27_30_26949 : Outport
  wires:
  Constant_-201.061929829747_e8334/1 -> Product_1c8cb/1
  Constant_376.991118430775_f2cd8/1 -> Product_1a1ae/1
  Product_1a1ae/1 -> Add_97ca2/2
  Product_1c8cb/1 -> Add_97ca2/1
  State_id_line_27_30_d82b5/1 -> Product_1c8cb/2
  State_iq_line_27_30_37807/1 -> Product_1a1ae/2
  Product_cd5ec/1 -> Add_96799/2
  Constant_628.318530717959_fb4b7/1 -> Product_cd5ec/1
  State_vd_bus_27_614b7/1 -> Product_cd5ec/2
  Add_97ca2/1 -> Add_96799/1
  Constant_628.318530717959_93a50/1 -> Product_7e1c1/1
  State_vd_bus_30_fc433/1 -> Product_7e1c1/2
  Add_96799/1 -> Subtract_78c91/1
  Product_7e1c1/1 -> Subtract_78c91/2
  Subtract_78c91/1 -> Blockout_d_id_line_27_30_26949/1

== system IEEE30_case/AC_1/d_id_line_28_27_block ==
  note: d_id_line_28_27 in IEEE30_case
      | $376.991118430775\,\mathrm{iq}_{\mathrm{line},28,27}-942.477796076938\,\mathrm{vd}_{\mathrm{bus},27}+942.477796076938\,\mathrm{vd}_{\mathrm{bus},28}$
      | Automatically generated on 2025-11-01 18:42:18 .
  State_iq_line_28_27_dccca : Inport
  State_vd_bus_27_3c49b : Inport  Port=2
  State_vd_bus_28_9edc3 : Inport  Port=3
  Add_5a52f : Sum
  Constant_376.991118430775_1fec1 : Constant  Value=376.991118430775
  Constant_942.477796076938_f8750 : Constant  Value=942.477796076938
  Constant_942.477796076938_fdf5b : Constant  Value=942.477796076938
  Product_2f72c : Product
  Product_b348e : Product
  Product_f548b : Product
  Subtract_0b23e : Sum  Inputs=+-
  Blockout_d_id_line_28_27_ed70c : Outport
  wires:
  Product_f548b/1 -> Subtract_0b23e/2
  Constant_376.991118430775_1fec1/1 -> Product_b348e/1
  State_iq_line_28_27_dccca/1 -> Product_b348e/2
  Product_b348e/1 -> Subtract_0b23e/1
  Constant_942.477796076938_fdf5b/1 -> Product_f548b/1
  State_vd_bus_27_3c49b/1 -> Product_f548b/2
  State_vd_bus_28_9edc3/1 -> Product_2f72c/2
  Product_2f72c/1 -> Add_5a52f/2
  Constant_942.477796076938_f8750/1 -> Product_2f72c/1
  Subtract_0b23e/1 -> Add_5a52f/1
  Add_5a52f/1 -> Blockout_d_id_line_28_27_ed70c/1

== system IEEE30_case/AC_1/d_id_line_29_30_block ==
  note: d_id_line_29_30 in IEEE30_case
      | $376.991118430775\,\mathrm{iq}_{\mathrm{line},29,30}-201.061929829747\,\mathrm{id}_{\mathrm{line},29,30}+837.758040957278\,\mathrm{vd}_{\mathrm{bus},29}-837.758040957278\,\mathrm{vd}_{\mathrm{bus},30}$
      | Automatically generated on 2025-11-01 18:42:25 .
  State_id_line_29_30_49020 : Inport
  State_iq_line_29_30_06255 : Inport  Port=2
  State_vd_bus_29_072b3 : Inport  Port=3
  State_vd_bus_30_f5954 : Inport  Port=4
  Add_0cb52 : Sum
  Add_d08ad : Sum
  Constant_-201.061929829747_5f060 : Constant  Value=-201.061929829747
  Constant_376.991118430775_295f6 : Constant  Value=376.991118430775
  Constant_837.758040957278_087ec : Constant  Value=837.758040957278
  Constant_837.758040957278_5bf06 : Constant  Value=837.758040957278
  Product_166c7 : Product
  Product_6a4ca : Product
  Product_74e3f : Product
  Product_ca41c : Product
  Subtract_90d91 : Sum  Inputs=+-
  Blockout_d_id_line_29_30_18eb7 : Outport
  wires:
  Constant_-201.061929829747_5f060/1 -> Product_ca41c/1
  State_id_line_29_30_49020/1 -> Product_ca41c/2
  Constant_376.991118430775_295f6/1 -> Product_74e3f/1
  State_iq_line_29_30_06255/1 -> Product_74e3f/2
  Product_ca41c/1 -> Add_0cb52/1
  Product_74e3f/1 -> Add_0cb52/2
  State_vd_bus_29_072b3/1 -> Product_6a4ca/2
  Product_6a4ca/1 -> Add_d08ad/2
  Constant_837.758040957278_087ec/1 -> Product_6a4ca/1
  Add_0cb52/1 -> Add_d08ad/1
  Product_166c7/1 -> Subtract_90d91/2
  Constant_837.758040957278_5bf06/1 -> Product_166c7/1
  State_vd_bus_30_f5954/1 -> Product_166c7/2
  Add_d08ad/1 -> Subtract_90d91/1
  Subtract_90d91/1 -> Blockout_d_id_line_29_30_18eb7/1

== system IEEE30_case/AC_1/d_id_line_2_4_block ==
  note: d_id_line_2_4 in IEEE30_case
      | $376.991118430775\,\mathrm{iq}_{\mathrm{line},2,4}-133.055688857921\,\mathrm{id}_{\mathrm{line},2,4}+2217.59481429868\,\mathrm{vd}_{\mathrm{bus},2}-2217.59481429868\,\mathrm{vd}_{\mathrm{bus},4}$
      | Automatically generated on 2025-11-01 18:41:01 .
  State_id_line_2_4_3a3db : Inport
  State_iq_line_2_4_7f64b : Inport  Port=2
  State_vd_bus_2_1a8e6 : Inport  Port=3
  State_vd_bus_4_468ae : Inport  Port=4
  Add_7126c : Sum
  Add_8abce : Sum
  Constant_-133.055688857921_51435 : Constant  Value=-133.055688857921
  Constant_2217.59481429868_a95a8 : Constant  Value=2217.59481429868
  Constant_2217.59481429868_e1024 : Constant  Value=2217.59481429868
  Constant_376.991118430775_6f80e : Constant  Value=376.991118430775
  Product_44319 : Product
  Product_50bac : Product
  Product_57253 : Product
  Product_de045 : Product
  Subtract_9bdad : Sum  Inputs=+-
  Blockout_d_id_line_2_4_f10ed : Outport
  wires:
  Constant_-133.055688857921_51435/1 -> Product_50bac/1
  Constant_376.991118430775_6f80e/1 -> Product_44319/1
  Product_44319/1 -> Add_7126c/2
  Product_50bac/1 -> Add_7126c/1
  State_id_line_2_4_3a3db/1 -> Product_50bac/2
  Subtract_9bdad/1 -> Blockout_d_id_line_2_4_f10ed/1
  State_iq_line_2_4_7f64b/1 -> Product_44319/2
  Product_de045/1 -> Add_8abce/2
  Constant_2217.59481429868_e1024/1 -> Product_de045/1
  State_vd_bus_2_1a8e6/1 -> Product_de045/2
  Add_7126c/1 -> Add_8abce/1
  Constant_2217.59481429868_a95a8/1 -> Product_57253/1
  State_vd_bus_4_468ae/1 -> Product_57253/2
  Add_8abce/1 -> Subtract_9bdad/1
  Product_57253/1 -> Subtract_9bdad/2

== system IEEE30_case/AC_1/d_id_line_2_5_block ==
  note: d_id_line_2_5 in IEEE30_case
      | $376.991118430775\,\mathrm{iq}_{\mathrm{line},2,5}-94.2477796076938\,\mathrm{id}_{\mathrm{line},2,5}+1884.95559215388\,\mathrm{vd}_{\mathrm{bus},2}-1884.95559215388\,\mathrm{vd}_{\mathrm{bus},5}$
      | Automatically generated on 2025-11-01 18:41:06 .
  State_id_line_2_5_56197 : Inport
  State_iq_line_2_5_6b567 : Inport  Port=2
  State_vd_bus_2_fba8e : Inport  Port=3
  State_vd_bus_5_3f7e8 : Inport  Port=4
  Add_03089 : Sum
  Add_68de3 : Sum
  Constant_-94.2477796076938_8f3fe : Constant  Value=-94.2477796076938
  Constant_1884.95559215388_11d12 : Constant  Value=1884.95559215388
  Constant_1884.95559215388_8a64f : Constant  Value=1884.95559215388
  Constant_376.991118430775_5c4e8 : Constant  Value=376.991118430775
  Product_01ac4 : Product
  Product_2b5e7 : Product
  Product_c3e8a : Product
  Product_cb634 : Product
  Subtract_25762 : Sum  Inputs=+-
  Blockout_d_id_line_2_5_534b8 : Outport
  wires:
  Subtract_25762/1 -> Blockout_d_id_line_2_5_534b8/1
  State_id_line_2_5_56197/1 -> Product_c3e8a/2
  Constant_-94.2477796076938_8f3fe/1 -> Product_c3e8a/1
  Constant_376.991118430775_5c4e8/1 -> Product_2b5e7/1
  Product_2b5e7/1 -> Add_68de3/2
  State_iq_line_2_5_6b567/1 -> Product_2b5e7/2
  Product_c3e8a/1 -> Add_68de3/1
  Constant_1884.95559215388_8a64f/1 -> Product_cb634/1
  State_vd_bus_2_fba8e/1 -> Product_cb634/2
  Add_68de3/1 -> Add_03089/1
  Product_cb634/1 -> Add_03089/2
  Product_01ac4/1 -> Subtract_25762/2
  Constant_1884.95559215388_11d12/1 -> Product_01ac4/1
  State_vd_bus_5_3f7e8/1 -> Product_01ac4/2
  Add_03089/1 -> Subtract_25762/1

== system IEEE30_case/AC_1/d_id_line_2_6_block ==
  note: d_id_line_2_6 in IEEE30_case
      | $376.991118430775\,\mathrm{iq}_{\mathrm{line},2,6}-125.663706143592\,\mathrm{id}_{\mathrm{line},2,6}+2094.39510239319\,\mathrm{vd}_{\mathrm{bus},2}-2094.39510239319\,\mathrm{vd}_{\mathrm{bus},6}$
      | Automatically generated on 2025-11-01 18:41:08 .
  State_id_line_2_6_7d8f0 : Inport
  State_iq_line_2_6_13ccb : Inport  Port=2
  State_vd_bus_2_83f23 : Inport  Port=3
  State_vd_bus_6_4e456 : Inport  Port=4
  Add_0c99a : Sum
  Add_987e2 : Sum
  Constant_-125.663706143592_70734 : Constant  Value=-125.663706143592
  Constant_2094.39510239319_abc6b : Constant  Value=2094.39510239319
  Constant_2094.39510239319_c8fe3 : Constant  Value=2094.39510239319
  Constant_376.991118430775_0a200 : Constant  Value=376.991118430775
  Product_164a9 : Product
  Product_60ae9 : Product
  Product_68e7d : Product
  Product_fed8f : Product
  Subtract_22aee : Sum  Inputs=+-
  Blockout_d_id_line_2_6_9ce60 : Outport
  wires:
  Constant_-125.663706143592_70734/1 -> Product_60ae9/1
  State_id_line_2_6_7d8f0/1 -> Product_60ae9/2
  Constant_376.991118430775_0a200/1 -> Product_68e7d/1
  Product_68e7d/1 -> Add_0c99a/2
  Product_164a9/1 -> Add_987e2/2
  Constant_2094.39510239319_c8fe3/1 -> Product_164a9/1
  Subtract_22aee/1 -> Blockout_d_id_line_2_6_9ce60/1
  State_iq_line_2_6_13ccb/1 -> Product_68e7d/2
  Product_60ae9/1 -> Add_0c99a/1
  State_vd_bus_2_83f23/1 -> Product_164a9/2
  Add_0c99a/1 -> Add_987e2/1
  Product_fed8f/1 -> Subtract_22aee/2
  Constant_2094.39510239319_abc6b/1 -> Product_fed8f/1
  Add_987e2/1 -> Subtract_22aee/1
  State_vd_bus_6_4e456/1 -> Product_fed8f/2

== system IEEE30_case/AC_1/d_id_line_3_4_block ==
  note: d_id_line_3_4 in IEEE30_case
      | $376.991118430775\,\mathrm{iq}_{\mathrm{line},3,4}-94.2477796076938\,\mathrm{id}_{\mathrm{line},3,4}+9424.77796076938\,\mathrm{vd}_{\mathrm{bus},3}-9424.77796076938\,\mathrm{vd}_{\mathrm{bus},4}$
      | Automatically generated on 2025-11-01 18:41:04 .
  State_id_line_3_4_c783d : Inport
  State_iq_line_3_4_97dfa : Inport  Port=2
  State_vd_bus_3_9cd0a : Inport  Port=3
  State_vd_bus_4_76476 : Inport  Port=4
  Add_3d560 : Sum
  Add_8be73 : Sum
  Constant_-94.2477796076938_018ba : Constant  Value=-94.2477796076938
  Constant_376.991118430775_93c8a : Constant  Value=376.991118430775
  Constant_9424.77796076938_35258 : Constant  Value=9424.77796076938
  Constant_9424.77796076938_e536f : Constant  Value=9424.77796076938
  Product_0b0d0 : Product
  Product_18d93 : Product
  Product_2ec61 : Product
  Product_9e69c : Product
  Subtract_27cbc : Sum  Inputs=+-
  Blockout_d_id_line_3_4_45374 : Outport
  wires:
  Constant_-94.2477796076938_018ba/1 -> Product_18d93/1
  Constant_376.991118430775_93c8a/1 -> Product_0b0d0/1
  State_id_line_3_4_c783d/1 -> Product_18d93/2
  Product_0b0d0/1 -> Add_8be73/2
  State_iq_line_3_4_97dfa/1 -> Product_0b0d0/2
  Product_9e69c/1 -> Add_3d560/2
  Constant_9424.77796076938_e536f/1 -> Product_9e69c/1
  Product_18d93/1 -> Add_8be73/1
  State_vd_bus_3_9cd0a/1 -> Product_9e69c/2
  Add_8be73/1 -> Add_3d560/1
  Product_2ec61/1 -> Subtract_27cbc/2
  Constant_9424.77796076938_35258/1 -> Product_2ec61/1
  State_vd_bus_4_76476/1 -> Product_2ec61/2
  Add_3d560/1 -> Subtract_27cbc/1
  Subtract_27cbc/1 -> Blockout_d_id_line_3_4_45374/1

== system IEEE30_case/AC_1/d_id_line_4_12_block ==
  note: d_id_line_4_12 in IEEE30_case
      | $376.991118430775\,\mathrm{iq}_{\mathrm{line},4,12}+1449.96584011837\,\mathrm{vd}_{\mathrm{bus},4}-1449.96584011837\,\mathrm{vd}_{\mathrm{bus},12}$
      | Automatically generated on 2025-11-01 18:41:29 .
  State_iq_line_4_12_530ed : Inport
  State_vd_bus_12_eb3f5 : Inport  Port=2
  State_vd_bus_4_83c34 : Inport  Port=3
  Add_52cce : Sum
  Constant_1449.96584011837_2b0bd : Constant  Value=1449.96584011837
  Constant_1449.96584011837_2baba : Constant  Value=1449.96584011837
  Constant_376.991118430775_f1dc3 : Constant  Value=376.991118430775
  Product_4dc9b : Product
  Product_a8af6 : Product
  Product_e1d6c : Product
  Subtract_23ed5 : Sum  Inputs=+-
  Blockout_d_id_line_4_12_f1df0 : Outport
  wires:
  Constant_376.991118430775_f1dc3/1 -> Product_4dc9b/1
  State_iq_line_4_12_530ed/1 -> Product_4dc9b/2
  Constant_1449.96584011837_2baba/1 -> Product_a8af6/1
  Product_a8af6/1 -> Subtract_23ed5/2
  State_vd_bus_12_eb3f5/1 -> Product_a8af6/2
  Product_4dc9b/1 -> Subtract_23ed5/1
  Constant_1449.96584011837_2b0bd/1 -> Product_e1d6c/1
  State_vd_bus_4_83c34/1 -> Product_e1d6c/2
  Subtract_23ed5/1 -> Add_52cce/1
  Product_e1d6c/1 -> Add_52cce/2
  Add_52cce/1 -> Blockout_d_id_line_4_12_f1df0/1

== system IEEE30_case/AC_1/d_id_line_4_6_block ==
  note: d_id_line_4_6 in IEEE30_case
      | $376.991118430775\,\mathrm{iq}_{\mathrm{line},4,6}-94.2477796076938\,\mathrm{id}_{\mathrm{line},4,6}+9424.77796076938\,\mathrm{vd}_{\mathrm{bus},4}-9424.77796076938\,\mathrm{vd}_{\mathrm{bus},6}$
      | Automatically generated on 2025-11-01 18:41:11 .
  State_id_line_4_6_53ca8 : Inport
  State_iq_line_4_6_0a7d7 : Inport  Port=2
  State_vd_bus_4_4594e : Inport  Port=3
  State_vd_bus_6_4e65f : Inport  Port=4
  Add_08850 : Sum
  Add_6ce23 : Sum
  Constant_-94.2477796076938_2c2f3 : Constant  Value=-94.2477796076938
  Constant_376.991118430775_df624 : Constant  Value=376.991118430775
  Constant_9424.77796076938_38598 : Constant  Value=9424.77796076938
  Constant_9424.77796076938_6b3a7 : Constant  Value=9424.77796076938
  Product_04022 : Product
  Product_5f21c : Product
  Product_a53a8 : Product
  Product_f8b36 : Product
  Subtract_b7fbd : Sum  Inputs=+-
  Blockout_d_id_line_4_6_c5916 : Outport
  wires:
  State_vd_bus_4_4594e/1 -> Product_5f21c/2
  Constant_-94.2477796076938_2c2f3/1 -> Product_f8b36/1
  Product_5f21c/1 -> Add_6ce23/2
  Constant_9424.77796076938_6b3a7/1 -> Product_5f21c/1
  Product_f8b36/1 -> Add_08850/1
  Subtract_b7fbd/1 -> Blockout_d_id_line_4_6_c5916/1
  State_id_line_4_6_53ca8/1 -> Product_f8b36/2
  Constant_376.991118430775_df624/1 -> Product_a53a8/1
  Product_a53a8/1 -> Add_08850/2
  State_iq_line_4_6_0a7d7/1 -> Product_a53a8/2
  Add_08850/1 -> Add_6ce23/1
  Constant_9424.77796076938_38598/1 -> Product_04022/1
  State_vd_bus_6_4e65f/1 -> Product_04022/2
  Add_6ce23/1 -> Subtract_b7fbd/1
  Product_04022/1 -> Subtract_b7fbd/2
